simulink model "E2"  (R2014a)
settings: Solver=ode45  StartTime=0.0  StopTime=40  RelTol=1e-3
values from neighbouring files (symbols this model uses):
  Kc = 800    [E01.m]
  Kr = 2    [E01.m]
libraries: cstblocks x1, simulink x1
settings Model: Creator=Davide  LastModifiedBy=Davide

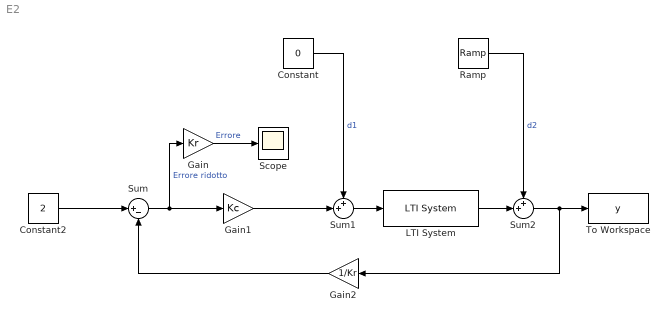
== system E2 ==
  Constant : Constant  Value=0
  Constant2 : Constant  Value=2
  Gain : Gain  Gain=Kr
  Gain1 : Gain  Gain=Kc
  Gain2 : Gain  Gain=1/Kr
  LTI System : cstblocks/LTI System  sys=F  IC=[]
  Ramp : simulink/Sources/Ramp  slope=0.01  start=0  X0=0
  Scope : Scope
  Sum : Sum  Inputs=|+-
  Sum1 : Sum  Inputs=++|
  Sum2 : Sum  Inputs=++|
  To Workspace : ToWorkspace  VariableName=y  SaveFormat=Timeseries  SampleTime=-1
  wires:
  Constant2/1 -> Sum/1
  Constant/1 -> Sum1/1  "d1"
  Sum/1 -> Gain/1, Gain1/1  "Errore ridotto"
  Sum1/1 -> LTI System/1
  LTI System/1 -> Sum2/2
  Ramp/1 -> Sum2/1  "d2"
  Sum2/1 -> Gain2/1, To Workspace/1
  Gain/1 -> Scope/1  "Errore"
  Gain1/1 -> Sum1/2
  Gain2/1 -> Sum/2
